simulink model "Simulator_Case_2"  (R2024a)
settings: Solver=VariableStepAuto  StartTime=0.0  StopTime=2800  RelTol=1e-3
values from neighbouring files (symbols this model uses):
  Desired_Year_IGRF = decyear('31-December-2024','dd-mmm-yyyy')    [Parametrization_Simulation_Case_2.m]
  Position_Initial_X = Waypoints_X(1)    [Parametrization_Simulation_Case_2.m]
  Position_Initial_Y = Waypoints_Y(1)    [Parametrization_Simulation_Case_2.m]
undefined symbols (not defined in the file or in its folder): Amplitude_Wave_Lake, Amplitude_Wind_Lake, Factor_Wave_1, Factor_Wave_2, Gain_Derivative_Controller, Gain_Integral_Controller, Gain_Proportional_Controller, Gain_Wind, Pulsation_Wave_Lake, Pulsation_Wind_Lake, Static_Gain_Waves, Time_Constant_Wind, Velocity_Ship_Mean, Waypoints
libraries: simulink_extras x4, cstblocks x2, simulink x2, sensorgpslib x1, sensorinslib x1
settings Model: Creator=gerar  LastModifiedBy=gerar
settings DebuggingCC: UnderSpecifiedDimensionMsg=warning

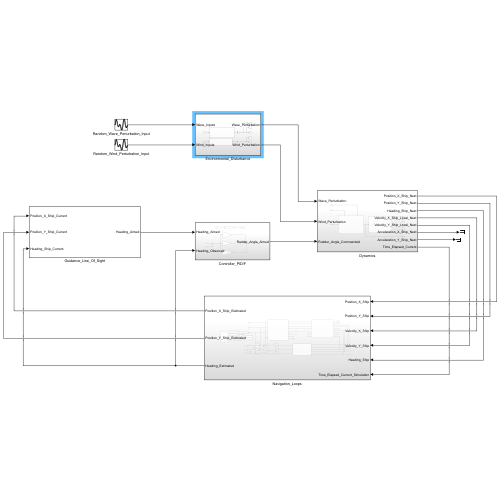
[thumbnail: Simulink's stored preview of the top-level diagram]
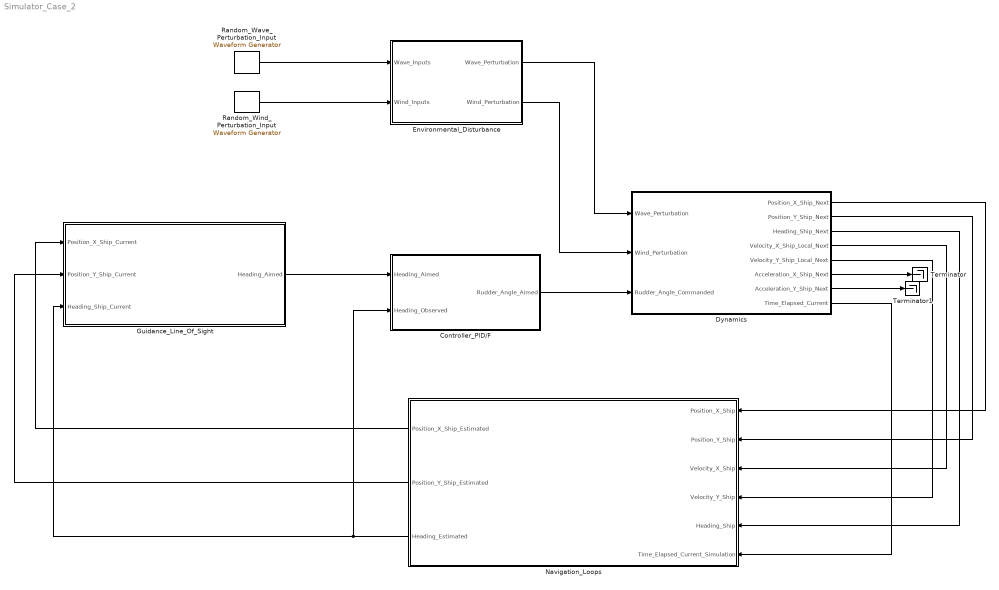
== system Simulator_Case_2 ==
  Controller_PID/F : Subsystem
  Dynamics : Subsystem
  Environmental_Disturbance : Subsystem
  Guidance_Line_Of_Sight : Subsystem
  Navigation_Loops : Subsystem
  Random_Wave_Perturbation_Input : simulink/Sources/Waveform Generator  OutMin=[]  OutMax=[]  OutDataTypeStr=double  SelectedSignal=1  Signals=sin(Amplitude_Wave_Lake, Pulsation_Wave_Lake, 1)  BlockNames=MultiportSwitch_d32ce6a50cc3442  SampleTime=0.1
  Random_Wind_Perturbation_Input : simulink/Sources/Waveform Generator  OutMin=[]  OutMax=[]  OutDataTypeStr=double  SelectedSignal=1  Signals=sin(Amplitude_Wind_Lake, Pulsation_Wind_Lake, 1)  BlockNames=MultiportSwitch_7513ca4c417b4ee  SampleTime=0.1
  Terminator : Terminator
  Terminator1 : Terminator
  wires:
  Random_Wave_Perturbation_Input/1 -> Environmental_Disturbance/1(Wave_Inputs)
  Guidance_Line_Of_Sight/1(Heading_Aimed) -> Controller_PID/F/1(Heading_Aimed)
  Random_Wind_Perturbation_Input/1 -> Environmental_Disturbance/2(Wind_Inputs)
  Environmental_Disturbance/1(Wave_Perturbation) -> Dynamics/1(Wave_Perturbation)
  Environmental_Disturbance/2(Wind_Perturbation) -> Dynamics/2(Wind_Perturbation)
  Controller_PID/F/1(Rudder_Angle_Aimed) -> Dynamics/3(Rudder_Angle_Commanded)
  Navigation_Loops/1(Position_X_Ship_Estimated) -> Guidance_Line_Of_Sight/1(Position_X_Ship_Current)
  Navigation_Loops/2(Position_Y_Ship_Estimated) -> Guidance_Line_Of_Sight/2(Position_Y_Ship_Current)
  Navigation_Loops/3(Heading_Estimated) -> Controller_PID/F/2(Heading_Observed), Guidance_Line_Of_Sight/3(Heading_Ship_Current)
  Dynamics/1(Position_X_Ship_Next) -> Navigation_Loops/1(Position_X_Ship)
  Dynamics/2(Position_Y_Ship_Next) -> Navigation_Loops/2(Position_Y_Ship)
  Dynamics/5(Velocity_Y_Ship_Local_Next) -> Navigation_Loops/4(Velocity_Y_Ship)
  Dynamics/8(Time_Elapsed_Current) -> Navigation_Loops/6(Time_Elapsed_Current_Simulation)
  Dynamics/6(Acceleration_X_Ship_Next) -> Terminator/1
  Dynamics/7(Acceleration_Y_Ship_Next) -> Terminator1/1
  Dynamics/3(Heading_Ship_Next) -> Navigation_Loops/5(Heading_Ship)
  Dynamics/4(Velocity_X_Ship_Local_Next) -> Navigation_Loops/3(Velocity_X_Ship)

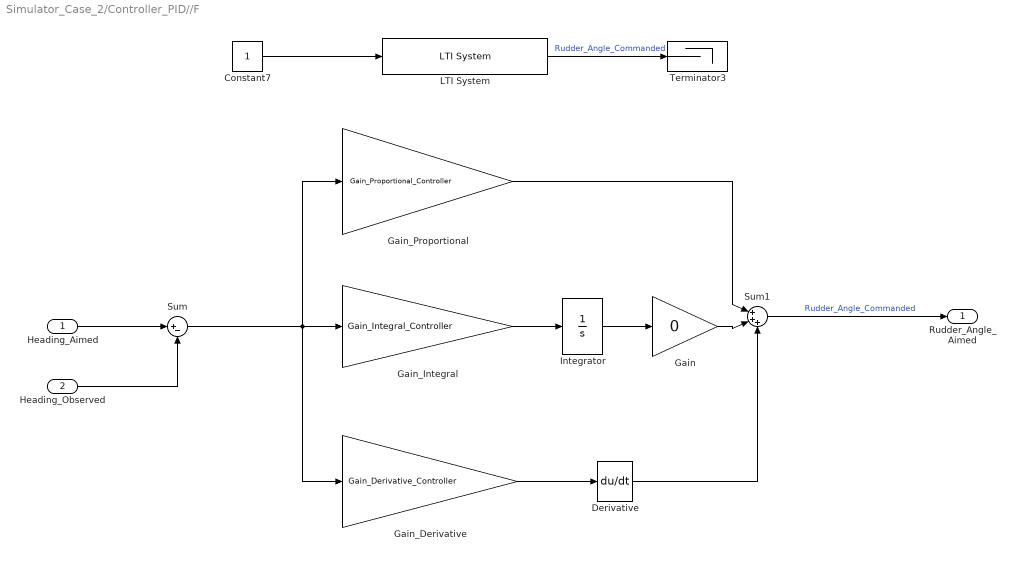
== system Simulator_Case_2/Controller_PID//F ==
  Heading_Aimed : Inport
  Heading_Observed : Inport  Port=2
  Constant7 : Constant
  Derivative : Derivative
  Gain : Gain  Gain=0
  Gain_Derivative : Gain  Gain=Gain_Derivative_Controller
  Gain_Integral : Gain  Gain=Gain_Integral_Controller
  Gain_Proportional : Gain  Gain=Gain_Proportional_Controller
  Integrator : Integrator  InitialCondition=-5*(pi/180)
  LTI System : cstblocks/LTI System  sys=Controller_PIDF  IC=[]  PadeOrder=0
  Sum : Sum  Inputs=|+-
  Sum1 : Sum  Inputs=|+++
  Terminator3 : Terminator
  Rudder_Angle_Aimed : Outport
  wires:
  Heading_Aimed/1 -> Sum/1
  Heading_Observed/1 -> Sum/2
  Sum1/1 -> Rudder_Angle_Aimed/1  "Rudder_Angle_Commanded"
  Gain_Proportional/1 -> Sum1/1
  Gain/1 -> Sum1/2
  Gain_Integral/1 -> Integrator/1
  Gain_Derivative/1 -> Derivative/1
  Derivative/1 -> Sum1/3
  Integrator/1 -> Gain/1
  Sum/1 -> Gain_Derivative/1, Gain_Integral/1, Gain_Proportional/1
  LTI System/1 -> Terminator3/1  "Rudder_Angle_Commanded"
  Constant7/1 -> LTI System/1

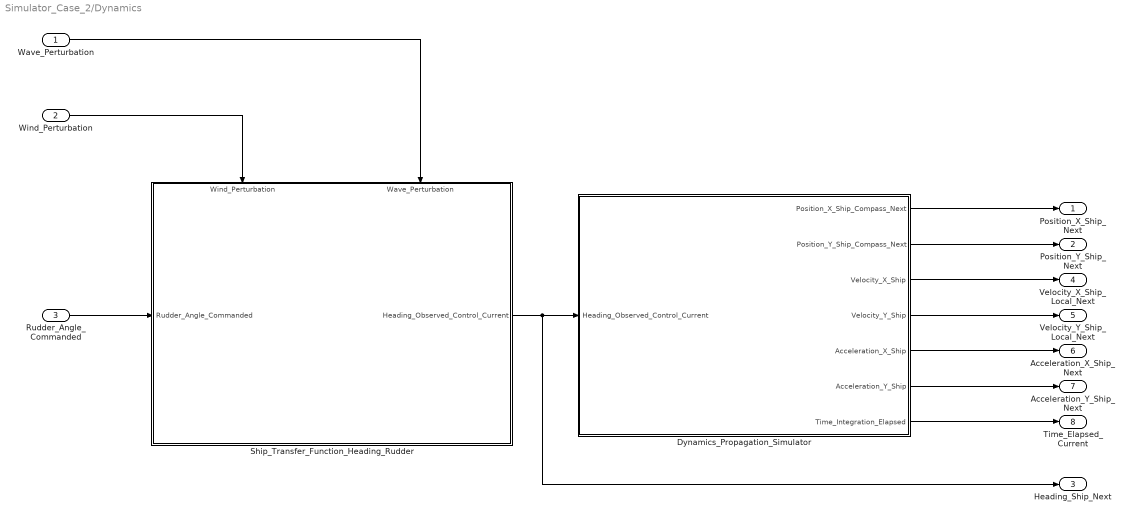
== system Simulator_Case_2/Dynamics ==
  Wave_Perturbation : Inport
  Wind_Perturbation : Inport  Port=2
  Rudder_Angle_Commanded : Inport  Port=3
  Dynamics_Propagation_Simulator : Subsystem
  Ship_Transfer_Function_Heading_Rudder : Subsystem
      settings: PortSchema="{\"entries\":[{\"content\":{\"sides\":[{\"content\":{\"connectorIds\":[\"In1\"]},\"type\":\"ConnectorPlacement.EquallySpacedRectSide\",\"uuid\":\"39a47681-8a87-4f22-9e16-0ead526089e0\"},{\"content\":{\"connectorIds\":[\"Out1\"],\"side\":\"RIGHT\"},\"type\":\"ConnectorPlacement.EquallySpacedRectSide\",\"uuid\":\"e7d068dc-643f-44db-a553-0a54b66f6b70\"},{\"content\":{\"connectorIds\":[\"In2\",\"In3\"],\"side\":\"TOP\"},\"type\":\"ConnectorPlacement.EquallySpacedRectSide\",\"uuid\":\"f984f23d-1b96-40dd-a354-9bced51babaa\"}]},\"type\":\"ConnectorPlacement.EquallySpacedConnector\",\"uuid\":\"30082198-c592-4bfc-a5f8-ae0235b1924b\"}],\"packageUris\":[\"http://schema.mathworks.com/mf0/Connector/R2020b\"],\"version\":\"1.0\"}"
  Position_X_Ship_Next : Outport
  Position_Y_Ship_Next : Outport  Port=2
  Heading_Ship_Next : Outport  Port=3
  Velocity_X_Ship_Local_Next : Outport  Port=4
  Velocity_Y_Ship_Local_Next : Outport  Port=5
  Acceleration_X_Ship_Next : Outport  Port=6
  Acceleration_Y_Ship_Next : Outport  Port=7
  Time_Elapsed_Current : Outport  Port=8
  wires:
  Ship_Transfer_Function_Heading_Rudder/1(Heading_Observed_Control_Current) -> Heading_Ship_Next/1, Dynamics_Propagation_Simulator/1(Heading_Observed_Control_Current)
  Wave_Perturbation/1 -> Ship_Transfer_Function_Heading_Rudder/3(Wave_Perturbation)
  Rudder_Angle_Commanded/1 -> Ship_Transfer_Function_Heading_Rudder/1(Rudder_Angle_Commanded)
  Dynamics_Propagation_Simulator/2(Position_Y_Ship_Compass_Next) -> Position_Y_Ship_Next/1
  Dynamics_Propagation_Simulator/4(Velocity_Y_Ship) -> Velocity_Y_Ship_Local_Next/1
  Wind_Perturbation/1 -> Ship_Transfer_Function_Heading_Rudder/2(Wind_Perturbation)
  Dynamics_Propagation_Simulator/5(Acceleration_X_Ship) -> Acceleration_X_Ship_Next/1
  Dynamics_Propagation_Simulator/1(Position_X_Ship_Compass_Next) -> Position_X_Ship_Next/1
  Dynamics_Propagation_Simulator/3(Velocity_X_Ship) -> Velocity_X_Ship_Local_Next/1
  Dynamics_Propagation_Simulator/6(Acceleration_Y_Ship) -> Acceleration_Y_Ship_Next/1
  Dynamics_Propagation_Simulator/7(Time_Integration_Elapsed) -> Time_Elapsed_Current/1

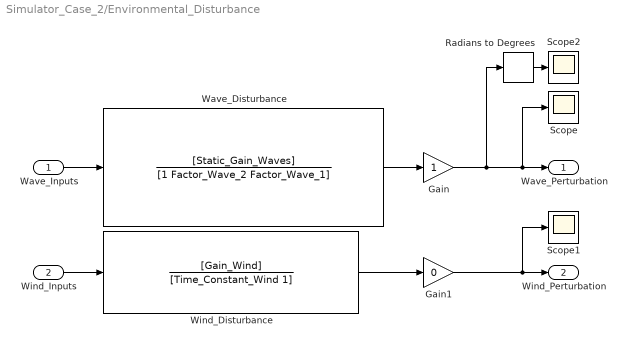
== system Simulator_Case_2/Environmental_Disturbance ==
  Wave_Inputs : Inport
  Wind_Inputs : Inport  Port=2
  Gain : Gain
  Gain1 : Gain  Gain=0
  Radians to Degrees : simulink_extras/Transformations/Radians to Degrees
  Scope : Scope
  Scope1 : Scope
  Scope2 : Scope
  Wave_Disturbance : TransferFcn  Numerator=[Static_Gain_Waves]  Denominator=[1 Factor_Wave_2 Factor_Wave_1]
  Wind_Disturbance : TransferFcn  Numerator=[Gain_Wind]  Denominator=[Time_Constant_Wind 1]
  Wave_Perturbation : Outport
  Wind_Perturbation : Outport  Port=2
  wires:
  Wind_Inputs/1 -> Wind_Disturbance/1
  Wave_Inputs/1 -> Wave_Disturbance/1
  Wind_Disturbance/1 -> Gain1/1
  Gain/1 -> Radians to Degrees/1, Scope/1, Wave_Perturbation/1
  Gain1/1 -> Scope1/1, Wind_Perturbation/1
  Wave_Disturbance/1 -> Gain/1
  Radians to Degrees/1 -> Scope2/1

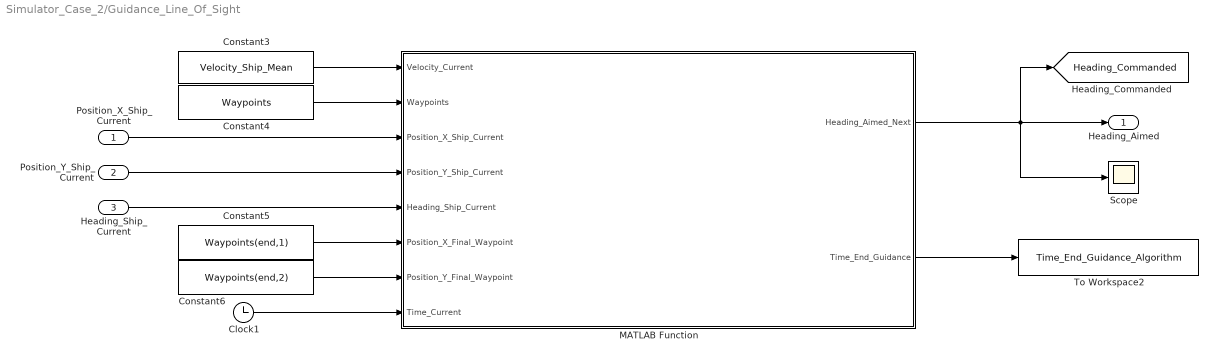
== system Simulator_Case_2/Guidance_Line_Of_Sight ==
  Position_X_Ship_Current : Inport
  Position_Y_Ship_Current : Inport  Port=2
  Heading_Ship_Current : Inport  Port=3
  Clock1 : Clock
  Constant3 : Constant  Value=Velocity_Ship_Mean
  Constant4 : Constant  Value=Waypoints
  Constant5 : Constant  Value=Waypoints(end,1)
  Constant6 : Constant  Value=Waypoints(end,2)
  MATLAB Function : MATLAB Function  TreatAsAtomicUnit=on
  Scope : Scope
  To Workspace2 : ToWorkspace  VariableName=Time_End_Guidance_Algorithm  SaveFormat=Timeseries  SampleTime=-1
  Heading_Aimed : Outport
  tag scope: Heading_Commanded=global
  wires:
  Constant5/1 -> MATLAB Function/6(Position_X_Final_Waypoint)
  Position_X_Ship_Current/1 -> MATLAB Function/3(Position_X_Ship_Current)
  MATLAB Function/1(Heading_Aimed_Next) -> Scope/1, [Heading_Commanded], Heading_Aimed/1
  Constant4/1 -> MATLAB Function/2(Waypoints)
  Constant3/1 -> MATLAB Function/1(Velocity_Current)
  Constant6/1 -> MATLAB Function/7(Position_Y_Final_Waypoint)
  Clock1/1 -> MATLAB Function/8(Time_Current)
  Position_Y_Ship_Current/1 -> MATLAB Function/4(Position_Y_Ship_Current)
  MATLAB Function/2(Time_End_Guidance) -> To Workspace2/1
  Heading_Ship_Current/1 -> MATLAB Function/5(Heading_Ship_Current)

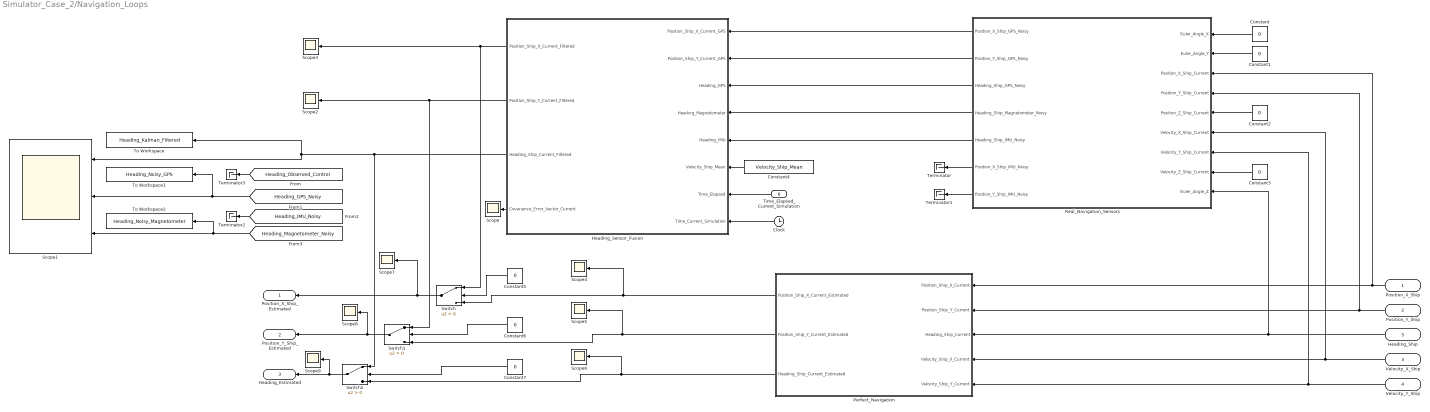
== system Simulator_Case_2/Navigation_Loops ==
  Position_X_Ship : Inport
  Position_Y_Ship : Inport  Port=2
  Velocity_X_Ship : Inport  Port=3
  Velocity_Y_Ship : Inport  Port=4
  Heading_Ship : Inport  Port=5
  Time_Elapsed_Current_Simulation : Inport  Port=6
  Clock : Clock
  Constant{,1..3,5..7} (7 alike) : Constant  Value=0
  Constant4 : Constant  Value=Velocity_Ship_Mean
  Heading_Sensor_Fusion : MATLAB Function  TreatAsAtomicUnit=on
  Perfect_Navigation : Subsystem
  Real_Navigation_Sensors : Subsystem
  Scope{,2..9} (9 alike) : Scope
  Scope1 : Scope  NumInputPorts=3
  Switch : Switch  Criteria=u2 > Threshold  SaturateOnIntegerOverflow=off  InputSameDT=off
  Switch1 : Switch  Criteria=u2 > Threshold  SaturateOnIntegerOverflow=off  InputSameDT=off
  Switch2 : Switch  Criteria=u2 > Threshold  SaturateOnIntegerOverflow=off  InputSameDT=off
  Terminator{,1..3} (4 alike) : Terminator
  To Workspace : ToWorkspace  VariableName=Heading_Kalman_Filtered  SaveFormat=Timeseries  SampleTime=-1
  To Workspace1 : ToWorkspace  VariableName=Heading_Noisy_GPS  SaveFormat=Timeseries  SampleTime=-1
  To Workspace2 : ToWorkspace  VariableName=Heading_Noisy_Magnetometer  SaveFormat=Timeseries  SampleTime=-1
  Position_X_Ship_Estimated : Outport
  Position_Y_Ship_Estimated : Outport  Port=2
  Heading_Estimated : Outport  Port=3
  wires:
  Position_X_Ship/1 -> Real_Navigation_Sensors/3(Position_X_Ship_Current), Perfect_Navigation/1(Position_Ship_X_Current)
  Position_Y_Ship/1 -> Real_Navigation_Sensors/4(Position_Y_Ship_Current), Perfect_Navigation/2(Position_Ship_Y_Current)
  Heading_Ship/1 -> Real_Navigation_Sensors/9(Euler_Angle_Z), Perfect_Navigation/3(Heading_Ship_Current)
  Velocity_X_Ship/1 -> Real_Navigation_Sensors/6(Velocity_X_Ship_Current), Perfect_Navigation/4(Velocity_Ship_X_Current)
  Velocity_Y_Ship/1 -> Real_Navigation_Sensors/7(Velocity_Y_Ship_Current), Perfect_Navigation/5(Velocity_Ship_Y_Current)
  Time_Elapsed_Current_Simulation/1 -> Heading_Sensor_Fusion/7(Time_Elapsed)
  Constant4/1 -> Heading_Sensor_Fusion/6(Velocity_Ship_Mean)
  Real_Navigation_Sensors/1(Position_X_Ship_GPS_Noisy) -> Heading_Sensor_Fusion/1(Position_Ship_X_Current_GPS)
  Real_Navigation_Sensors/2(Position_Y_Ship_GPS_Noisy) -> Heading_Sensor_Fusion/2(Position_Ship_Y_Current_GPS)
  Real_Navigation_Sensors/3(Heading_Ship_GPS_Noisy) -> Heading_Sensor_Fusion/3(Heading_GPS)
  Real_Navigation_Sensors/4(Heading_Ship_Magnetometer_Noisy) -> Heading_Sensor_Fusion/4(Heading_Magnetometer)
  Real_Navigation_Sensors/5(Heading_Ship_IMU_Noisy) -> Heading_Sensor_Fusion/5(Heading_IMU)
  Real_Navigation_Sensors/6(Position_X_Ship_IMU_Noisy) -> Terminator/1
  Real_Navigation_Sensors/7(Position_Y_Ship_IMU_Noisy) -> Terminator1/1
  Heading_Sensor_Fusion/4(Covariance_Error_Vector_Current) -> Scope/1
  Heading_Sensor_Fusion/2(Position_Ship_Y_Current_Filtered) -> Switch1/1, Scope2/1
  Heading_Sensor_Fusion/1(Position_Ship_X_Current_Filtered) -> Switch/1, Scope3/1
  Heading_Sensor_Fusion/3(Heading_Ship_Current_Filtered) -> Switch2/1, To Workspace/1, Scope1/1
  Constant/1 -> Real_Navigation_Sensors/1(Euler_Angle_X)
  Constant1/1 -> Real_Navigation_Sensors/2(Euler_Angle_Y)
  Constant2/1 -> Real_Navigation_Sensors/5(Position_Z_Ship_Current)
  Constant3/1 -> Real_Navigation_Sensors/8(Velocity_Z_Ship_Current)
  Clock/1 -> Heading_Sensor_Fusion/8(Time_Current_Simulation)
  [Heading_GPS_Noisy] -> To Workspace1/1, Scope1/2
  [Heading_Magnetometer_Noisy] -> To Workspace2/1, Scope1/3
  [Heading_IMU_Noisy] -> Terminator2/1
  [Heading_Observed_Control] -> Terminator3/1
  Perfect_Navigation/1(Position_Ship_X_Current_Estimated) -> Scope4/1, Switch/3
  Constant5/1 -> Switch/2
  Switch/1 -> Position_X_Ship_Estimated/1, Scope7/1
  Perfect_Navigation/2(Position_Ship_Y_Current_Estimated) -> Scope5/1, Switch1/3
  Constant6/1 -> Switch1/2
  Switch1/1 -> Scope8/1, Position_Y_Ship_Estimated/1
  Switch2/1 -> Scope9/1, Heading_Estimated/1
  Perfect_Navigation/3(Heading_Ship_Current_Estimated) -> Scope6/1, Switch2/3
  Constant7/1 -> Switch2/2

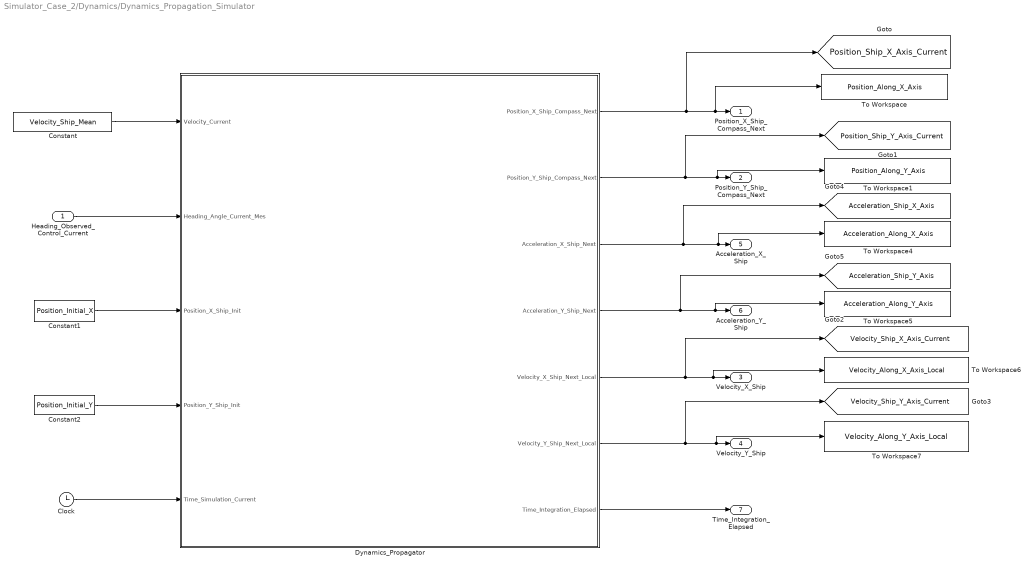
== system Simulator_Case_2/Dynamics/Dynamics_Propagation_Simulator ==
  Heading_Observed_Control_Current : Inport
  Clock : Clock
  Constant : Constant  Value=Velocity_Ship_Mean
  Constant1 : Constant  Value=Position_Initial_X
  Constant2 : Constant  Value=Position_Initial_Y
  Dynamics_Propagator : MATLAB Function  TreatAsAtomicUnit=on
  To Workspace : ToWorkspace  VariableName=Position_Along_X_Axis  SaveFormat=Timeseries  SampleTime=-1
  To Workspace1 : ToWorkspace  VariableName=Position_Along_Y_Axis  SaveFormat=Timeseries  SampleTime=-1
  To Workspace4 : ToWorkspace  VariableName=Acceleration_Along_X_Axis  SaveFormat=Timeseries  SampleTime=-1
  To Workspace5 : ToWorkspace  VariableName=Acceleration_Along_Y_Axis  SaveFormat=Timeseries  SampleTime=-1
  To Workspace6 : ToWorkspace  VariableName=Velocity_Along_X_Axis_Local  SaveFormat=Timeseries  SampleTime=-1
  To Workspace7 : ToWorkspace  VariableName=Velocity_Along_Y_Axis_Local  SaveFormat=Timeseries  SampleTime=-1
  Position_X_Ship_Compass_Next : Outport
  Position_Y_Ship_Compass_Next : Outport  Port=2
  Velocity_X_Ship : Outport  Port=3
  Velocity_Y_Ship : Outport  Port=4
  Acceleration_X_Ship : Outport  Port=5
  Acceleration_Y_Ship : Outport  Port=6
  Time_Integration_Elapsed : Outport  Port=7
  tag scope: Acceleration_Ship_X_Axis=global, Acceleration_Ship_Y_Axis=global, Position_Ship_X_Axis_Current=global, Position_Ship_Y_Axis_Current=global, Velocity_Ship_X_Axis_Current=global, Velocity_Ship_Y_Axis_Current=global
  wires:
  Heading_Observed_Control_Current/1 -> Dynamics_Propagator/2(Heading_Angle_Current_Mes)
  Constant/1 -> Dynamics_Propagator/1(Velocity_Current)
  Constant1/1 -> Dynamics_Propagator/3(Position_X_Ship_Init)
  Constant2/1 -> Dynamics_Propagator/4(Position_Y_Ship_Init)
  Clock/1 -> Dynamics_Propagator/5(Time_Simulation_Current)
  Dynamics_Propagator/1(Position_X_Ship_Compass_Next) -> Position_X_Ship_Compass_Next/1, To Workspace/1, [Position_Ship_X_Axis_Current]
  Dynamics_Propagator/2(Position_Y_Ship_Compass_Next) -> [Position_Ship_Y_Axis_Current], Position_Y_Ship_Compass_Next/1, To Workspace1/1
  Dynamics_Propagator/3(Acceleration_X_Ship_Next) -> [Acceleration_Ship_X_Axis], Acceleration_X_Ship/1, To Workspace4/1
  Dynamics_Propagator/4(Acceleration_Y_Ship_Next) -> [Acceleration_Ship_Y_Axis], Acceleration_Y_Ship/1, To Workspace5/1
  Dynamics_Propagator/5(Velocity_X_Ship_Next_Local) -> [Velocity_Ship_X_Axis_Current], Velocity_X_Ship/1, To Workspace6/1
  Dynamics_Propagator/6(Velocity_Y_Ship_Next_Local) -> [Velocity_Ship_Y_Axis_Current], Velocity_Y_Ship/1, To Workspace7/1
  Dynamics_Propagator/7(Time_Integration_Elapsed) -> Time_Integration_Elapsed/1

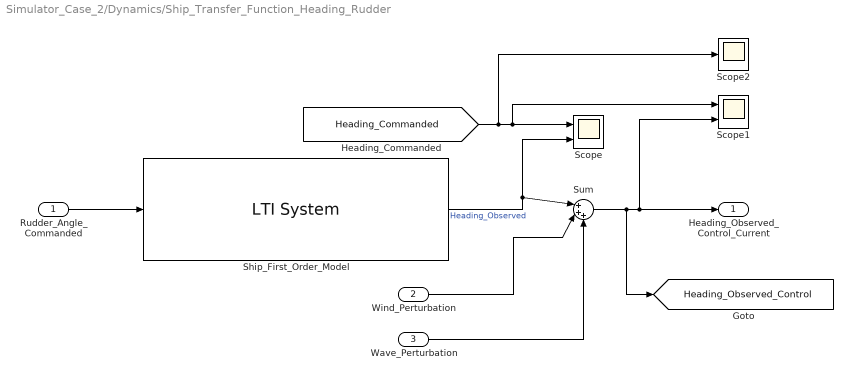
== system Simulator_Case_2/Dynamics/Ship_Transfer_Function_Heading_Rudder ==
  Rudder_Angle_Commanded : Inport
  Wind_Perturbation : Inport  Port=2
  Wave_Perturbation : Inport  Port=3
  Scope : Scope  NumInputPorts=2
  Scope1 : Scope  NumInputPorts=2
  Scope2 : Scope
  Ship_First_Order_Model : cstblocks/LTI System  sys=Heading_On_Rudder_Transfer_First_Order  IC=[]  PadeOrder=0
  Sum : Sum  Inputs=|+++
  Heading_Observed_Control_Current : Outport
  tag scope: Heading_Observed_Control=global
  wires:
  Ship_First_Order_Model/1 -> Scope/2, Sum/1  "Heading_Observed"
  Rudder_Angle_Commanded/1 -> Ship_First_Order_Model/1
  [Heading_Commanded] -> Scope2/1, Scope1/1, Scope/1
  Sum/1 -> [Heading_Observed_Control], Scope1/2, Heading_Observed_Control_Current/1
  Wind_Perturbation/1 -> Sum/2
  Wave_Perturbation/1 -> Sum/3

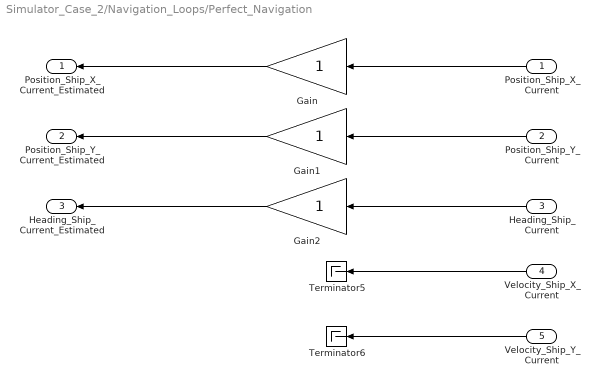
== system Simulator_Case_2/Navigation_Loops/Perfect_Navigation ==
  Position_Ship_X_Current : Inport
  Position_Ship_Y_Current : Inport  Port=2
  Heading_Ship_Current : Inport  Port=3
  Velocity_Ship_X_Current : Inport  Port=4
  Velocity_Ship_Y_Current : Inport  Port=5
  Gain : Gain
  Gain1 : Gain
  Gain2 : Gain
  Terminator5 : Terminator
  Terminator6 : Terminator
  Position_Ship_X_Current_Estimated : Outport
  Position_Ship_Y_Current_Estimated : Outport  Port=2
  Heading_Ship_Current_Estimated : Outport  Port=3
  wires:
  Position_Ship_X_Current/1 -> Gain/1
  Heading_Ship_Current/1 -> Gain2/1
  Gain2/1 -> Heading_Ship_Current_Estimated/1
  Gain/1 -> Position_Ship_X_Current_Estimated/1
  Velocity_Ship_Y_Current/1 -> Terminator6/1
  Velocity_Ship_X_Current/1 -> Terminator5/1
  Position_Ship_Y_Current/1 -> Gain1/1
  Gain1/1 -> Position_Ship_Y_Current_Estimated/1

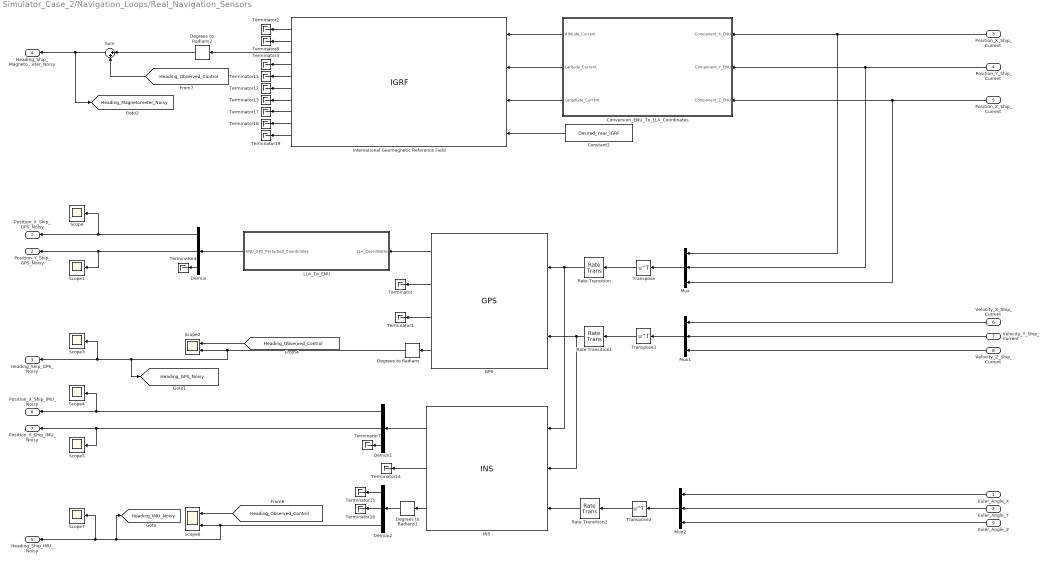
== system Simulator_Case_2/Navigation_Loops/Real_Navigation_Sensors ==
  Euler_Angle_X : Inport
  Euler_Angle_Y : Inport  Port=2
  Position_X_Ship_Current : Inport  Port=3
  Position_Y_Ship_Current : Inport  Port=4
  Position_Z_Ship_Current : Inport  Port=5
  Velocity_X_Ship_Current : Inport  Port=6
  Velocity_Y_Ship_Current : Inport  Port=7
  Velocity_Z_Ship_Current : Inport  Port=8
  Euler_Angle_Z : Inport  Port=9
  Constant2 : Constant  Value=Desired_Year_IGRF
  Conversion_ENU_To_LLA_Coordinates : MATLAB Function  TreatAsAtomicUnit=on
  Degrees to Radians : simulink_extras/Transformations/Degrees to Radians
  Degrees to Radians1 : simulink_extras/Transformations/Degrees to Radians
  Degrees to Radians2 : simulink_extras/Transformations/Degrees to Radians
  Demux : Demux  Outputs=3
  Demux1 : Demux  Outputs=3
  Demux2 : Demux  Outputs=3
  GPS : sensorgpslib/GPS  DispRefFrame=ENU  PositionInputFormat=Local  ReferenceLocation=[43.059023, 3.002915 ,0]  HorizontalPositionAccuracy=2  VerticalPositionAccuracy=2  VelocityAccuracy=0.1  DecayFactor=0.999  SeedDouble=67  SimulateUsing=Interpreted execution
  INS : sensorinslib/INS  MountingLocation=[0 0 0]  RollAccuracy=0.2  PitchAccuracy=0.2  YawAccuracy=1  PositionAccuracy=1  VelocityAccuracy=0.05  UseAccelAndAngVel=off  AccelerationAccuracy=0  AngularVelocityAccuracy=0  TimeInput=off  PositionErrorFactor=[0 0 0]  SeedDouble=67  SimulateUsing=Code generation
  International Geomagnetic Reference Field : IGRF  month=January  day=1  year=2020
      settings: AttributesFormatString=%<generation>
  LLA_To_ENU : MATLAB Function  TreatAsAtomicUnit=on
  Mux : Mux  Inputs=3
  Mux1 : Mux  Inputs=3
  Mux2 : Mux  Inputs=3
  Rate Transition : RateTransition  OutPortSampleTime=0.01
  Rate Transition1 : RateTransition  OutPortSampleTime=0.01
  Rate Transition2 : RateTransition  OutPortSampleTime=0.01
  Scope{,1,3..5,7} (6 alike) : Scope
  Scope2 : Scope  NumInputPorts=2
  Scope6 : Scope  NumInputPorts=2
  Sum : Sum  Inputs=|++
  Terminator{,1..4,7..8,11..19} (16 alike) : Terminator
  Transpose : Math  Operator=transpose
  Transpose1 : Math  Operator=transpose
  Transpose2 : Math  Operator=transpose
  Position_X_Ship_GPS_Noisy : Outport
  Position_Y_Ship_GPS_Noisy : Outport  Port=2
  Heading_Ship_GPS_Noisy : Outport  Port=3
  Heading_Ship_Magnetometer_Noisy : Outport  Port=4
  Heading_Ship_IMU_Noisy : Outport  Port=5
  Position_X_Ship_IMU_Noisy : Outport  Port=6
  Position_Y_Ship_IMU_Noisy : Outport  Port=7
  tag scope: Heading_GPS_Noisy=global, Heading_IMU_Noisy=global, Heading_Magnetometer_Noisy=global
  wires:
  [Heading_Observed_Control] -> Scope2/1
  INS/1 -> Demux1/1
  International Geomagnetic Reference Field/1 -> Terminator2/1
  Demux2/3 -> [Heading_IMU_Noisy], Heading_Ship_IMU_Noisy/1, Scope7/1, Scope6/2
  Position_Y_Ship_Current/1 -> Mux/2, Conversion_ENU_To_LLA_Coordinates/2(Component_Y_ENU)
  GPS/3 -> Terminator1/1
  International Geomagnetic Reference Field/6 -> Terminator12/1
  International Geomagnetic Reference Field/10 -> Terminator19/1
  Demux2/2 -> Terminator16/1
  Euler_Angle_X/1 -> Mux2/1
  Demux1/1 -> Position_X_Ship_IMU_Noisy/1, Scope4/1
  INS/2 -> Terminator14/1
  Demux/2 -> Position_Y_Ship_GPS_Noisy/1, Scope1/1
  [Heading_Observed_Control] -> Scope6/1
  International Geomagnetic Reference Field/5 -> Terminator11/1
  Degrees to Radians/1 -> [Heading_GPS_Noisy], Heading_Ship_GPS_Noisy/1, Scope3/1, Scope2/2
  Velocity_Y_Ship_Current/1 -> Mux1/2
  Rate Transition2/1 -> INS/3
  Conversion_ENU_To_LLA_Coordinates/1(Altitude_Current) -> International Geomagnetic Reference Field/1
  Demux2/1 -> Terminator15/1
  Demux/3 -> Terminator4/1
  Degrees to Radians2/1 -> Sum/1
  Mux2/1 -> Transpose2/1
  Mux/1 -> Transpose/1
  Demux1/3 -> Terminator7/1
  Position_X_Ship_Current/1 -> Mux/1, Conversion_ENU_To_LLA_Coordinates/1(Component_X_ENU)
  [Heading_Observed_Control] -> Sum/2
  Constant2/1 -> International Geomagnetic Reference Field/4
  Degrees to Radians1/1 -> Demux2/1
  INS/3 -> Degrees to Radians1/1
  GPS/4 -> Degrees to Radians/1
  Transpose2/1 -> Rate Transition2/1
  Demux1/2 -> Position_Y_Ship_IMU_Noisy/1, Scope5/1
  GPS/2 -> Terminator/1
  International Geomagnetic Reference Field/4 -> Terminator3/1
  Rate Transition1/1 -> INS/2, GPS/2
  Demux/1 -> Position_X_Ship_GPS_Noisy/1, Scope/1
  International Geomagnetic Reference Field/8 -> Terminator17/1
  International Geomagnetic Reference Field/2 -> Terminator8/1
  Transpose1/1 -> Rate Transition1/1
  Conversion_ENU_To_LLA_Coordinates/2(Latitude_Current) -> International Geomagnetic Reference Field/2
  Transpose/1 -> Rate Transition/1
  Rate Transition/1 -> INS/1, GPS/1
  Position_Z_Ship_Current/1 -> Mux/3, Conversion_ENU_To_LLA_Coordinates/3(Component_Z_ENU)
  Euler_Angle_Y/1 -> Mux2/2
  LLA_To_ENU/1(ENU_GPS_Perturbed_Coordinates) -> Demux/1
  Mux1/1 -> Transpose1/1
  International Geomagnetic Reference Field/3 -> Degrees to Radians2/1
  GPS/1 -> LLA_To_ENU/1(LLA_Coordinates)
  Conversion_ENU_To_LLA_Coordinates/3(Longitude_Current) -> International Geomagnetic Reference Field/3
  International Geomagnetic Reference Field/7 -> Terminator13/1
  International Geomagnetic Reference Field/9 -> Terminator18/1
  Velocity_Z_Ship_Current/1 -> Mux1/3
  Velocity_X_Ship_Current/1 -> Mux1/1
  Euler_Angle_Z/1 -> Mux2/3
  Sum/1 -> [Heading_Magnetometer_Noisy], Heading_Ship_Magnetometer_Noisy/1

== matlab function Simulator_Case_2/Navigation_Loops/Heading_Sensor_Fusion ==
  settings: updateMethod=DISCRETE
  data: Position_Ship_X_Current_GPS input; Position_Ship_Y_Current_GPS input; Heading_GPS input; Heading_Magnetometer input; Heading_IMU input; Position_Ship_X_Current_Filtered output; Position_Ship_Y_Current_Filtered output; Heading_Ship_Current_Filtered output; Covariance_Error_Vector_Current output; Velocity_Ship_Mean input; Time_Elapsed input; Time_Current_Simulation input
function [Position_Ship_X_Current_Filtered,...
          Position_Ship_Y_Current_Filtered,...
          Heading_Ship_Current_Filtered,...
          Covariance_Error_Vector_Current]  = Navigation_Kalman_Sensor_Fusion(Position_Ship_X_Current_GPS,...
                                                                              Position_Ship_Y_Current_GPS,...
                                                                              Heading_GPS,...
                                                                              Heading_Magnetometer,...
                                                                              Heading_IMU,...
                                                                              Velocity_Ship_Mean,...
                                                                              Time_Elapsed,...
                                                                              Time_Current_Simulation)

% This function serves as a filterting and data fusion to provide the ship
% with the right heading data.

persistent State_Model_Prediction;
persistent Covariance_Model_Prediction;

% Openwork modifications:
% - Include the position given by the IMU if needed.
% - Complexification of the state model.

% ----------------------------------------------------------------
% 1) Definition of the process model:
% ----------------------------------------------------------------
% We define the following process model state vector:
% States_Initial_Model = [Position_X_Current;...
%                   Position_Y_Current;...
%                   Psi_Heading_Current;...
%                   Velocity_Current];

% Initialization of the current models:
Position_Ship_X_Current_Model = Position_Ship_X_Current_GPS;
Position_Ship_Y_Current_Model = Position_Ship_Y_Current_GPS;
Heading_Current_Model = Heading_Magnetometer;
Velocity_Ship_Model = Velocity_Ship_Mean;

States_Initial_Model = [Position_Ship_X_Current_Model;...
                        Position_Ship_Y_Current_Model;...
                        Heading_Current_Model;...
                        Velocity_Ship_Model];

% We then define the process noise covariance matrix refered as the 'Q'
% matrix in estimation. This has a link with how one is confident about the
% used model:
Variance_Position_X = 5;
Variance_Position_Y = 5;
Variance_Heading = (15*pi/180);
Variance_Velocity = 0.5;
Process_Model_Covariance_Matrix = [Variance_Position_X^2 0 0 0;
                                   0 Variance_Position_Y^2 0 0;
                                   0 0 Variance_Heading^2 0;
                                   0 0 0 Variance_Velocity^2];

% We define the covariance matrix of the states at the initial step refered as the 'P0|0':
% We just take Covariance_Matrix_States_Initial_Model =
% Process_Model_Covariance_Matrix:
Covariance_States_Initial_Model = Process_Model_Covariance_Matrix;

% Define the control input matrix refered as the 'B' matrix in the usual
% description of linear state-space system reprezentation:
Control_Inputs_Initial = 0; % Process model considered as without input influence.

% Chose the step time, it shall be aligned with HW specification:
Time_Step_Integration = Time_Elapsed;

% NOTA:
% When calling the EKF function such that Estimates = EKF(), to get the
% proper evaluated functions used inside (Jacobians for example), then use
% the notation Estimates = EKF(Jacobian(Variable1,Variable2)).
% If it's not working, then delete the function as an input of the EKF,
% call it directly inside the EKF function. But pay attention to get the
% good inputs inside the EKF function.
% /!\ Same thing for the Function_Process_Model inside the EKF /!\.

% ----------------------------------------------------------------
% 2) Measurement & Innovation model:
% ----------------------------------------------------------------
% We define the following measurement model state vector:
% Measurement_Vector = [Position_X_Current;...
%                       Position_Y_Current;...
%                       Psi_Heading_GNSS_Current;...
%                       Psi_Heading_Mag_Current;...
%                       Psi_Heading_IMU_Current
%                       Velocity_Current];

% Definition of the measurement noise covariance matrix refered as 'R' matrix:
% Retake the Variance_Position_X, Variance_Position_Y, Variance_Velocity
% and Variance_Heading for Variance_Heading_GNSS used in the process model section:
% To be aligned with the specification from the sensors and the models used
% for the Navigation:
Variance_Position_X_GPS = 2;
Variance_Position_Y_GPS = 2;
Variance_Heading_GNSS = 2*(pi/180);
Variance_Heading_Magnetic = 2*(pi/180);
Variance_Velocity_Sensors = 0.1;
% Variance_Heading_IMU = 20*(pi/180);
% Measurement_Covariance_Matrix = [Variance_Position_X_GPS 0 0 0 0 0;
%                                  0 Variance_Position_Y_GPS 0 0 0 0;
%                                  0 0 Variance_Heading_GNSS 0 0 0;
%                                  0 0 0 Variance_Heading_Magnetic 0 0;
%                                  0 0 0 0 Variance_Heading_IMU 0;
%                                  0 0 0 0 0 Variance_Velocity];
Measurement_Covariance_Matrix = [Variance_Position_X_GPS 0 0 0 0;
                                 0 Variance_Position_Y_GPS 0 0 0;
                                 0 0 Variance_Heading_GNSS 0 0;
                                 0 0 0 Variance_Heading_Magnetic 0;
                                 0 0 0 0 Variance_Velocity_Sensors];

% Define the measurement model matrix: (ofter refered as 'H' or 'Gx'
% matrices):
% Measurement_Model_Matrix = [1 0 0 0;
%                             0 1 0 0;
%                             0 0 1 0;
%                             0 0 1 0;
%                             0 0 1 0;
%                             0 0 0 1];
Measurement_Model_Matrix = [1 0 0 0;
                            0 1 0 0;
                            0 0 1 0;
                            0 0 1 0;
                            0 0 0 1];


% ----------------------------------------------------------------
% Extended Kalman Filter loop calculations:
% ----------------------------------------------------------------
% Store the results:
% States_Estimated_EKF = [];
% Covariance_Estimated_EKF = [];

% Initialization:
if isempty(State_Model_Prediction)
    State_Model_Prediction = States_Initial_Model;
end
States_Previous = State_Model_Prediction; % The 'X' state vector.
if isempty(Covariance_Model_Prediction)
    Covariance_Model_Prediction = Covariance_States_Initial_Model;
end
Covariance_State_Previous = Covariance_Model_Prediction; % The 'P0|0' equal to 'Q' in this case.
Control_Inputs_Previous = Control_Inputs_Initial; % The usual 'B' matrix but unused here.
Process_Model_Covariance_Matrix_Previous = Process_Model_Covariance_Matrix; % The 'Q' process model matrix.
Measurement_Covariance_Matrix_Previous = Measurement_Covariance_Matrix; % The 'R' measurement matrix.
% Measurment_Current = [Position_Ship_X_Current_GPS,Position_Ship_Y_Current_GPS,Heading_GPS,Heading_Magnetometer,...
%                       Heading_IMU,Velocity_Ship_Mean];
Measurment_Current = [Position_Ship_X_Current_GPS,Position_Ship_Y_Current_GPS,Heading_GPS,Heading_Magnetometer,Velocity_Ship_Mean];

% EKF loop calculation:
[State_Aposteriori_Current,Covariance_Aposteriori_Current] = EKF_Heading(States_Previous,Covariance_State_Previous,Control_Inputs_Previous,...
                                                                         Jacobian_State_Process_Model(States_Previous(4),States_Previous(3),Time_Step_Integration),...
                                                                         Process_Model_Covariance_Matrix_Previous,Measurement_Model_Matrix,...
                                                                         Measurement_Covariance_Matrix_Previous,...
                                                                         Function_Process_Model(States_Previous(1),States_Previous(2),States_Previous(3),States_Previous(4),Time_Step_Integration),...
                                                                         Measurment_Current');


% Inputs update:
State_Model_Prediction = State_Aposteriori_Current; % This must be stored and reused at the next step time.
Covariance_Model_Prediction = Covariance_Aposteriori_Current;

% Store the interesting components of the covariance matrix (diagonal
% terms):
Covariance_Position_X = Covariance_Aposteriori_Current(1,1);
Covariance_Position_Y = Covariance_Aposteriori_Current(2,2);
Covariance_Psi_Heading = Covariance_Aposteriori_Current(3,3);
Covariance_Velocity = Covariance_Aposteriori_Current(4,4);
Covariance_Error_Vector_Current = [Covariance_Position_X;...
                                   Covariance_Position_Y;...
                                   Covariance_Psi_Heading;...
                                   Covariance_Velocity];

% Filtered and fused data:
Position_Ship_X_Current_Filtered = State_Aposteriori_Current(1);
Position_Ship_Y_Current_Filtered = State_Aposteriori_Current(2);
Heading_Ship_Current_Filtered = State_Aposteriori_Current(3);
Velocity_Current_Filtered = State_Aposteriori_Current(4); % The velocity is supposed constant.

end

== matlab function Simulator_Case_2/Guidance_Line_Of_Sight/MATLAB Function ==
  settings: updateMethod=DISCRETE
  data: Velocity_Current input; Heading_Aimed_Next output; Waypoints input; Position_X_Ship_Current input; Position_Y_Ship_Current input; Heading_Ship_Current input; Position_X_Final_Waypoint input; Position_Y_Final_Waypoint input; Time_Current input; Time_End_Guidance output
function [Heading_Aimed_Next,Time_End_Guidance] = Guidance_Waypoints_Following(Velocity_Current,...
                                                                               Waypoints,...
                                                                               Position_X_Ship_Current,...
                                                                               Position_Y_Ship_Current,...
                                                                               Heading_Ship_Current,...
                                                                               Position_X_Final_Waypoint,...
                                                                               Position_Y_Final_Waypoint,...
                                                                               Time_Current)

% Terminal point features:
Position_X_Final_Point = Position_X_Final_Waypoint;
Position_Y_Final_Point = Position_Y_Final_Waypoint;
Radius_Final_Waypoint = 50;
Heading_Error_Guidance_Activation = 5*(pi/180);

% Define persistent for heading protection:
persistent Heading_Previous;
if isempty(Heading_Previous)
    Heading_Previous = Heading_Ship_Current;
end

% Enable Guidance to work if the ship is not close to the final waypoint:
if ~((Position_X_Ship_Current - Position_X_Final_Point)^2 + (Position_Y_Ship_Current - Position_Y_Final_Point)^2 <= Radius_Final_Waypoint^2)

    % Then settle the time of end Guidance:
    Time_End_Guidance = 0;

    % Retreive the aimed heading angle that must be performed at this step time
    % of the simulation to follow the Waypoints generated trajectory:
    [Heading_Aimed_Unit,Heading_Aimed_Compass,...
     Heading_Error_Unit,Heading_Error_Compass,...
     Selected_Waypoints,Heading_Current_Unit] = Guidance_Heading_Rudder_Angle(Waypoints,...
                                                                              Position_X_Ship_Current,...
                                                                              Position_Y_Ship_Current, ...
                                                                              Heading_Ship_Current);

    % Update the heading aimed if an only if the heading error is greater
    % than a specified threshold:
    % Heading_Error = Heading_Aimed_Compass - Heading_Ship_Current;
    % if abs(Heading_Error) > Heading_Error_Guidance_Activation
    %     Heading_Aimed_Next = Heading_Aimed_Compass; % Update the Guidance command.
    % else
    %     Heading_Aimed_Next = Heading_Ship_Current; % Propagate the current state.
    % end
    Heading_Aimed_Next = Heading_Aimed_Compass;

    % Protection for the heading:
    if abs(Heading_Aimed_Next - Heading_Previous) > 150*(pi/180)
        Heading_Aimed_Next = Heading_Previous;
    end

    % Then update the persistent:
    Heading_Previous = Heading_Aimed_Next;       

else
    
    [Heading_Aimed_Unit,Heading_Aimed_Compass,...
     Heading_Error_Unit,Heading_Error_Compass,...
     Selected_Waypoints,Heading_Current_Unit] = Guidance_Heading_Rudder_Angle(Waypoints,...
                                                                              Position_X_Ship_Current,...
                                                                              Position_Y_Ship_Current, ...
                                                                              Heading_Ship_Current);

    % Update the heading aimed if an only if the heading error is greater
    % than a specified threshold:
    % Heading_Error = Heading_Aimed_Compass - Heading_Ship_Current;
    % if abs(Heading_Error) > Heading_Error_Guidance_Activation
    %     Heading_Aimed_Next = Heading_Aimed_Compass; % Update the Guidance command.
    % else
    %     Heading_Aimed_Next = Heading_Ship_Current; % Propagate the current state.
    % end
    Heading_Aimed_Next = Heading_Aimed_Compass;

    % Protection for the heading:
    if abs(Heading_Aimed_Next - Heading_Previous) > 40*(pi/180)
        Heading_Aimed_Next = Heading_Previous;
    end

    % Then update the persistent:
    Heading_Previous = Heading_Aimed_Next; 
    
    % Then determine the end time of the Guidance scheme:
    Time_End_Guidance = Time_Current;

end
end

== matlab function Simulator_Case_2/Dynamics/Dynamics_Propagation_Simulator/Dynamics_Propagator ==
  settings: updateMethod=DISCRETE
  data: Velocity_Current input; Heading_Angle_Current_Mes input; Position_X_Ship_Init input; Position_Y_Ship_Init input; Time_Simulation_Current input; Position_X_Ship_Compass_Next output; Position_Y_Ship_Compass_Next output; Acceleration_X_Ship_Next output; Acceleration_Y_Ship_Next output; Velocity_X_Ship_Next_Local output; Velocity_Y_Ship_Next_Local output; Time_Integration_Elapsed output
function [Position_X_Ship_Compass_Next,Position_Y_Ship_Compass_Next,...
          Acceleration_X_Ship_Next,Acceleration_Y_Ship_Next,...
          Velocity_X_Ship_Next_Local,Velocity_Y_Ship_Next_Local,Time_Integration_Elapsed] = Dynamics_Propagation(Velocity_Current,Heading_Angle_Current_Mes,...
                                                                                                                 Position_X_Ship_Init,Position_Y_Ship_Init,...
                                                                                                                 Time_Simulation_Current)

% Persistents definition:
persistent Position_X_Ship_Compass_Prev
persistent Position_Y_Ship_Compass_Prev
persistent Time_Simulation_Previous
persistent Heading_Previous
persistent Velocity_X_Ship_Local_Previous
persistent Velocity_Y_Ship_Local_Previous

% Heading previous storage:
if isempty(Heading_Previous)
    Heading_Previous = Heading_Angle_Current_Mes;
    Heading_Current = Heading_Previous;
else
    Heading_Current = Heading_Angle_Current_Mes;
end

% Simulation time handeling persistent:
if isempty(Time_Simulation_Previous)
    Time_Simulation_Previous = Time_Simulation_Current;
    Time_Integration_Elapsed = Time_Simulation_Current - Time_Simulation_Previous;
else
    Time_Integration_Elapsed = Time_Simulation_Current - Time_Simulation_Previous;
end
Time_Simulation_Previous = Time_Simulation_Current;

% Calculate the local position increment but use both convention (unit and compass):
% Compass:
Position_X_Ship_Current_Increment_Compass = Time_Integration_Elapsed*Velocity_Current*sin(Heading_Previous);
Position_Y_Ship_Current_Increment_Compass = Time_Integration_Elapsed*Velocity_Current*cos(Heading_Previous);

% The simple velocity discrete increment:
Velocity_X_Ship_Local = Velocity_Current*sin(Heading_Angle_Current_Mes);
Velocity_Y_Ship_Local = Velocity_Current*cos(Heading_Angle_Current_Mes);

if isempty(Velocity_X_Ship_Local_Previous)
    Velocity_X_Ship_Local_Previous = Velocity_Current*sin(Heading_Angle_Current_Mes);
    Acceleration_X_Ship_Next = 0;
else
    Acceleration_X_Ship_Next = (Velocity_X_Ship_Local - Velocity_X_Ship_Local_Previous)/Time_Integration_Elapsed;
    Velocity_X_Ship_Local_Previous = Velocity_X_Ship_Local;
end
if isempty(Velocity_Y_Ship_Local_Previous)
    Velocity_Y_Ship_Local_Previous = Velocity_Current*cos(Heading_Angle_Current_Mes);
    Acceleration_Y_Ship_Next = 0;
else
    Acceleration_Y_Ship_Next = (Velocity_Y_Ship_Local - Velocity_Y_Ship_Local_Previous)/Time_Integration_Elapsed;
    Velocity_Y_Ship_Local_Previous = Velocity_Y_Ship_Local;
end


% Compass position persistent filling:
if isempty(Position_X_Ship_Compass_Prev)
    Position_X_Ship_Compass_Prev = Position_X_Ship_Init + Position_X_Ship_Current_Increment_Compass;
else
    Position_X_Ship_Compass_Prev = Position_X_Ship_Compass_Prev + Position_X_Ship_Current_Increment_Compass;
end
if isempty(Position_Y_Ship_Compass_Prev)
    Position_Y_Ship_Compass_Prev = Position_Y_Ship_Init + Position_Y_Ship_Current_Increment_Compass;
else
    Position_Y_Ship_Compass_Prev = Position_Y_Ship_Compass_Prev + Position_Y_Ship_Current_Increment_Compass;
end

% Then update the outputs:
% Compass:
Position_X_Ship_Compass_Next = Position_X_Ship_Compass_Prev;
Position_Y_Ship_Compass_Next = Position_Y_Ship_Compass_Prev;

% Store the heading:
Heading_Estimated_Next = Heading_Current;
Heading_Previous = Heading_Estimated_Next;

% Velocity:
Velocity_X_Ship_Next_Local = Velocity_X_Ship_Local;
Velocity_Y_Ship_Next_Local = Velocity_Y_Ship_Local;

end

== matlab function Simulator_Case_2/Navigation_Loops/Real_Navigation_Sensors/LLA_To_ENU ==
  data: LLA_Coordinates input; ENU_GPS_Perturbed_Coordinates output
function ENU_GPS_Perturbed_Coordinates = Conversion_LLA_To_ENU(LLA_Coordinates)

% Reference point:
Reference_Point_Port_Mahon = [43.059023,3.002915,0];
Semi_Major_Axis = 6378137.0;
Flattening = 1/298.25;

% This function serves as a mean to convert LLA coordinates to ENU
% coordinates:
ENU_GPS_Perturbed_Coordinates = LLA_To_ENU(LLA_Coordinates(1),LLA_Coordinates(2),LLA_Coordinates(3),...
                                           Reference_Point_Port_Mahon(1),Reference_Point_Port_Mahon(2),...
                                           Reference_Point_Port_Mahon(3),Semi_Major_Axis,Flattening);


end

== matlab function Simulator_Case_2/Navigation_Loops/Real_Navigation_Sensors/Conversion_ENU_To_LLA_Coordinates ==
  data: Altitude_Current output; Latitude_Current output; Longitude_Current output; Component_X_ENU input; Component_Y_ENU input; Component_Z_ENU input
function [Altitude_Current,Latitude_Current,Longitude_Current] = Conversion_ENU_To_LAA(Component_X_ENU,...
                                                                                       Component_Y_ENU,...
                                                                                       Component_Z_ENU)

% This function serves as a mean to convert ENU coordinates into LLA
% coordinates. Need to write an embedded function to be injected in the
% Mission Software.
% Reference point for the current mission;
Reference_Point_Port_Mahon = [43.059023,3.002915,0];
Position_Vector_ENU_Current = [Component_X_ENU,Component_Y_ENU,Component_Z_ENU];

% Conversion using Matlab function:
Position_Vector_LLA_Current = enu2lla(Position_Vector_ENU_Current,Reference_Point_Port_Mahon,'ellipsoid');

% Feed the outputs:
Latitude_Current = Position_Vector_LLA_Current(1);
Altitude_Current = Position_Vector_LLA_Current(3);
Longitude_Current = Position_Vector_LLA_Current(2);

end
